simulink model "lab2_s"  (R2022b)
settings: Solver=ode23t  StartTime=0.0  StopTime=0.1  MaxStep=1e-5  RelTol=1e-3
values from neighbouring files (symbols this model uses):
  A = [-Ra/La -psi/La;psi/J 0]    [lab2_m.m]
  B = [1/La 0;0 -1/J]    [lab2_m.m]
  C = [0 1]    [lab2_m.m]
  D = [0 0]    [lab2_m.m]
  J = J2    (= 0.001501)    [lab2_m.m]
  La = 3.5e-4    (= 0.00035)    [lab2_m.m]
  psi = 0.229183    [lab2_m.m]
  Ra = 0.35    [lab2_m.m]
  T_L = 0    [lab2_m.m]
  U = U_rated    (= 24)    [lab2_m.m]
libraries: fl_lib x7, nesl_utility x5, ee_lib x1
settings Model: Creator=86156  LastModifiedBy=86156

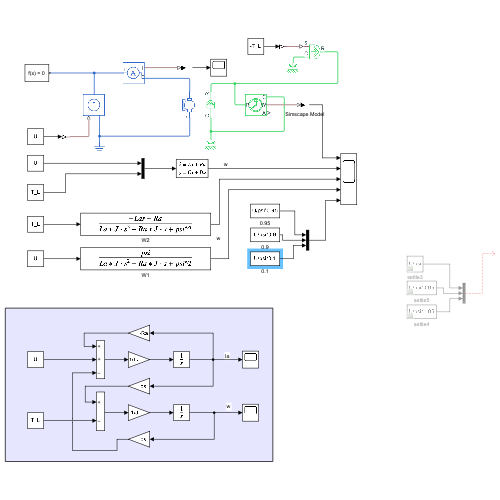
[thumbnail: Simulink's stored preview of the top-level diagram]
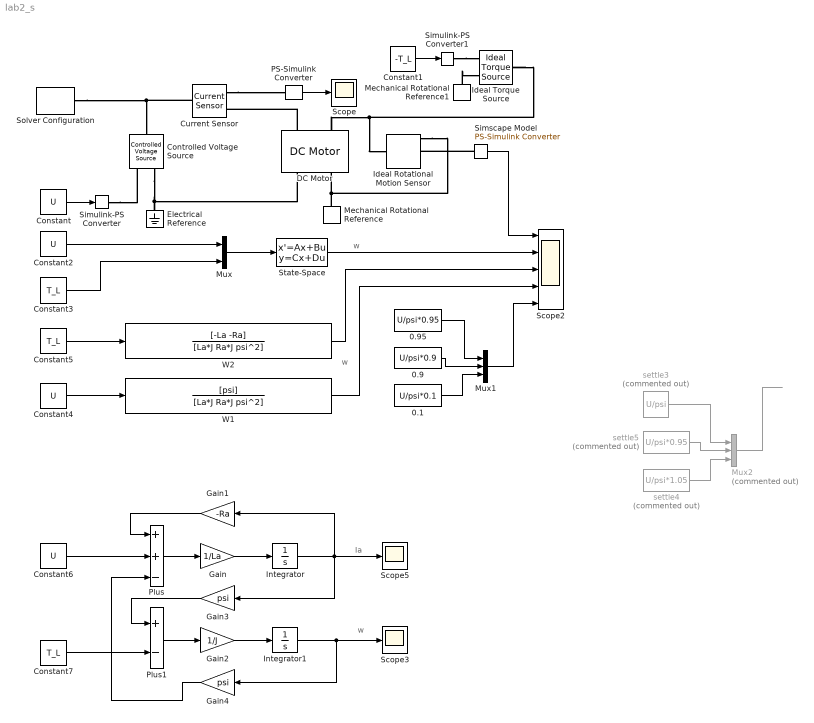
== system lab2_s ==
  note: Ia
  note: w
  note: w
  note: w
  0.1 : Constant  Value=U/psi*0.1
  0.9 : Constant  Value=U/psi*0.9
  0.95 : Constant  Value=U/psi*0.95
  Constant{,2,4,6} (4 alike) : Constant  Value=U
  Constant1 : Constant  Value=-T_L
  Constant3 : Constant  Value=T_L
  Constant5 : Constant  Value=T_L
  Constant7 : Constant  Value=T_L
  Controlled Voltage Source : fl_lib/Electrical/Electrical Sources/Controlled Voltage Source
  Current Sensor : fl_lib/Electrical/Electrical Sensors/Current Sensor
  DC Motor : ee_lib/Electromechanical/Brushed Motors/DC Motor  field_option=ee.enum.field_option.pm  Rf=100 Ohm  Lf=1 H  Laf=0.15 H  If0=0 A  parameterization=ee.enum.dcparam_option.circuit_param  Ra=Ra Ohm  La=La H  emf_or_torque=ee.enum.emf_or_torque.kv  Kv=psi V/(rad/s)  Ki=6.876e-4 N*m/A  T_stall=0.24e-3 N*m  w_max=19100 rpm  w_rated=15000 rpm  P_rated=0.08 W  V_rated=1.5 V  lam_param=ee.enum.lam_param.damping  i_noload=0 A  V_i_noload=1.5 V  J=J kg*m^2  lam=0 N*m/(rad/s)  speed0=0 rpm  enable_fault_armature=simscape.enum.onoff.off  rev_faulted=1 / 3  G_faulted_armature=1e-5 S  fault_trigger_armature=ee.enum.faults.faultTrigger.temporal  t_fault_armature=1 s  max_permissible_current_armature=inf A  t_fail_on_current_armature=1 s  enable_fault_field=simscape.enum.onoff.off  G_faulted_field=1e-5 S  fault_trigger_field=ee.enum.faults.faultTrigger.temporal  t_fault_field=1 s  max_permissible_current_field=inf A  t_fail_on_current_field=1 s  fault_action=simscape.enum.assert.action.none  alpha=3.93e-3 1/K  Tmeas=25 degC  thermal_mass=100 J/K  initial_temperature=25 degC
  Electrical Reference : fl_lib/Electrical/Electrical Elements/Electrical Reference
  Gain : Gain  Gain=1/La
  Gain1 : Gain  Gain=-Ra
  Gain2 : Gain  Gain=1/J
  Gain3 : Gain  Gain=psi
  Gain4 : Gain  Gain=psi
  Ideal Rotational Motion Sensor : fl_lib/Mechanical/Mechanical Sensors/Ideal Rotational Motion Sensor  reference=foundation.enum.MeasurementReference.difference  acceleration_port=false  velocity_port=true  position_port=true  wrap_angle=false  offset=0 rad
  Ideal Torque Source : fl_lib/Mechanical/Mechanical Sources/Ideal Torque Source
  Integrator : Integrator
  Integrator1 : Integrator
  Mechanical Rotational Reference : fl_lib/Mechanical/Rotational Elements/Mechanical Rotational Reference
  Mechanical Rotational Reference1 : fl_lib/Mechanical/Rotational Elements/Mechanical Rotational Reference
  Mux : Mux  Inputs=2
  Mux1 : Mux  Inputs=3
  Mux2 : Mux  Commented=on  Inputs=3
  PS-Simulink Converter : nesl_utility/PS-Simulink Converter  PhysicalDomain=network_engine_domain  SubClassName=ps_output  LeftPortType=input  RightPortType=output  PseudoPeriodic=off  Frequencies=[]  VectorFormat=inherit  Unit=inherit  AffineConversion=off
  Plus : Sum  Inputs=++-
  Plus1 : Sum  Inputs=+-
  Scope : Scope
  Scope2 : Scope  NumInputPorts=5
  Scope3 : Scope
  Scope5 : Scope
  Simscape Model : nesl_utility/PS-Simulink Converter  PhysicalDomain=network_engine_domain  SubClassName=ps_output  LeftPortType=input  RightPortType=output  PseudoPeriodic=off  Frequencies=[]  VectorFormat=inherit  Unit=inherit  AffineConversion=off
  Simulink-PS Converter : nesl_utility/Simulink-PS Converter  PhysicalDomain=network_engine_domain  SubClassName=ps_input  LeftPortType=input  RightPortType=output  PseudoPeriodic=off  Frequencies=[]  NoiseDistribution=none  NoiseParameters=[]  Unit=1  AffineConversion=off  FilteringAndDerivatives=provide  SimscapeFilterOrder=1  InputFilterTimeConstant=0.001  UdotUserProvided=0
  Simulink-PS Converter1 : nesl_utility/Simulink-PS Converter  PhysicalDomain=network_engine_domain  SubClassName=ps_input  LeftPortType=input  RightPortType=output  PseudoPeriodic=off  Frequencies=[]  NoiseDistribution=none  NoiseParameters=[]  Unit=1  AffineConversion=off  FilteringAndDerivatives=provide  SimscapeFilterOrder=1  InputFilterTimeConstant=0.001  UdotUserProvided=0
  Solver Configuration : nesl_utility/Solver Configuration  PhysicalDomain=network_engine_domain  SubClassName=solver  LeftPortType=input  RightPortType=generic  Tones=[]  Harmonics=[]  SimulateNoise=off  Profile=off  UseLocalSampling=off  EnableSwitchedLinearOptims=on  FrequencyDomain=off  UseCCode=off  RelTol=0.001  AbsTol=0.001  MinStep=1e-09  ToWorkspace=off  RevertToSquareIcSolve=off  NumHomotopyIterations=100  PhasorMode=off  PhasorModeNumHarmonics=1  ConsistencySolver=NEWTON_XTOL_AFTER_FTOL  IndexReductionMethod=DerivativeReplacement  DoDC=off  ResidualTolerance=1e-09  ConsistencyTolSource=GLOBAL  ConsistencyAbsTol=0.001  ConsistencyRelTol=0.001  ConsistencyTolFactor=0.001  UseLocalSolver=off  LocalSolverChoice=NE_BACKWARD_EULER_ADVANCER  ResolveIndetEquations=on  FunctionEvalNumThread=1  LocalSolverSampleTime=0.001  DoFixedCost=off  MaxNonlinIter=3  MaxModeIter=2  ComputeImpulses=off  ImpulseIterations=2  LinearAlgebra=auto  LinearAlgebraNumThread=0  EquationFormulation=NE_TIME_EF  DelaysMemoryBudget=1024  AutomaticFiltering=on  FilteringTimeConstant=0.001  PartitionStorageMethod=AS_NEEDED  PartitionMemoryBudget=1024  PartitionMethod=ROBUST
  State-Space : StateSpace  A=A  B=B  C=C  D=D  InitialCondition=0
  W1 : TransferFcn  Numerator=[psi]  Denominator=[La*J Ra*J psi^2]
  W2 : TransferFcn  Numerator=[-La -Ra]  Denominator=[La*J Ra*J psi^2]
  settle3 : Constant  Commented=on  Value=U/psi
  settle4 : Constant  Commented=on  Value=U/psi*1.05
  settle5 : Constant  Commented=on  Value=U/psi*0.95
  wires:
  Constant/1 -> Simulink-PS Converter/1
  PS-Simulink Converter/1 -> Scope/1
  Constant1/1 -> Simulink-PS Converter1/1
  Simscape Model/1 -> Scope2/1
  Constant2/1 -> Mux/1
  Constant3/1 -> Mux/2
  Mux/1 -> State-Space/1
  State-Space/1 -> Scope2/2
  Constant4/1 -> W1/1
  Constant5/1 -> W2/1
  W2/1 -> Scope2/3
  Constant6/1 -> Plus/2
  Plus/1 -> Gain/1
  Gain/1 -> Integrator/1
  Gain1/1 -> Plus/1
  Constant7/1 -> Plus1/2
  Plus1/1 -> Gain2/1
  Integrator/1 -> Gain3/1, Scope5/1, Gain1/1
  Gain3/1 -> Plus1/1
  Gain2/1 -> Integrator1/1
  Gain4/1 -> Plus/3
  Integrator1/1 -> Scope3/1, Gain4/1
  W1/1 -> Scope2/4
  0.9/1 -> Mux1/2
  0.1/1 -> Mux1/3
  Mux1/1 -> Scope2/5
  settle5/1 -> Mux2/2
  Mux2/1 -> ?
  settle3/1 -> Mux2/1
  settle4/1 -> Mux2/3
  0.95/1 -> Mux1/1
  connections:
  Simulink-PS Converter/RConn1 -- Controlled Voltage Source/RConn1
  Solver Configuration/RConn1 -- Controlled Voltage Source/LConn1 -- Current Sensor/LConn1
  Current Sensor/RConn1 -- PS-Simulink Converter/LConn1
  Controlled Voltage Source/RConn2 -- Electrical Reference/LConn1 -- DC Motor/RConn1
  DC Motor/LConn1 -- Current Sensor/RConn2
  Mechanical Rotational Reference/LConn1 -- Ideal Rotational Motion Sensor/RConn1 -- DC Motor/RConn2
  DC Motor/LConn2 -- Ideal Torque Source/LConn1 -- Ideal Rotational Motion Sensor/LConn1
  Simscape Model/LConn1 -- Ideal Rotational Motion Sensor/RConn2
  Simulink-PS Converter1/RConn1 -- Ideal Torque Source/RConn1
  Mechanical Rotational Reference1/LConn1 -- Ideal Torque Source/RConn2
